simulink model "dis_ut"  (Simulink 8.1)
settings: Solver=ode45  StartTime=0.0  StopTime=10.0  RelTol=1e-3
libraries: siltestlib x4, dis x1
settings Model: Creator=xsellart  LastModifiedBy=AT015555
settings DataIOCC: SignalLoggingSaveFormat=Dataset
settings OptimizationCC: ExpressionDepthLimit=128
settings DebuggingCC: FcnCallInpInsideContextMsg=EnableAllAsError
settings GRTTargetCC: CombineOutputUpdateFcns=on  GRTInterface=off

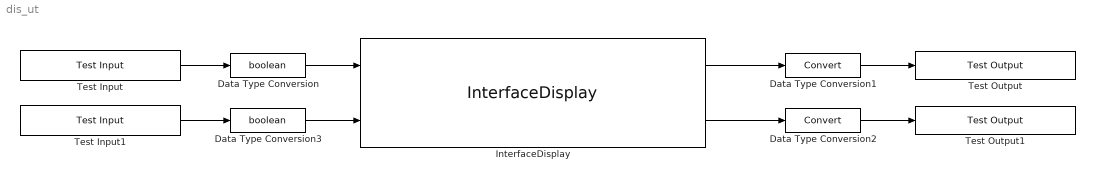
== system dis_ut ==
  Data Type Conversion : DataTypeConversion  OutDataTypeStr=boolean
  Data Type Conversion1 : DataTypeConversion
  Data Type Conversion2 : DataTypeConversion
  Data Type Conversion3 : DataTypeConversion  OutDataTypeStr=boolean
  InterfaceDisplay : dis/InterfaceDisplay
  Test Input : siltestlib/Test Input  varname=VDINR_FCWEnabledHMI_flg  sampletime=-1
  Test Input1 : siltestlib/Test Input  varname=VDINR_AEBEnabledHMI_flg  sampletime=-1
  Test Output : siltestlib/Test Output  varname=VIFO_FCWDisabledViaHMI_flg  sampletime=-1
  Test Output1 : siltestlib/Test Output  varname=VIFO_AEBDisabledViaHMI_flg  sampletime=-1
  wires:
  InterfaceDisplay/1 -> Data Type Conversion1/1
  Data Type Conversion1/1 -> Test Output/1
  InterfaceDisplay/2 -> Data Type Conversion2/1
  Data Type Conversion2/1 -> Test Output1/1
  Test Input/1 -> Data Type Conversion/1
  Data Type Conversion/1 -> InterfaceDisplay/1
  Test Input1/1 -> Data Type Conversion3/1
  Data Type Conversion3/1 -> InterfaceDisplay/2
